simulink model "zad1b"  (R2016a)
settings: Solver=ode5  StartTime=0.0  StopTime=20  FixedStep=0.01  RelTol=1e-3
values from neighbouring files (symbols this model uses):
  b = 3    [zad1script.m]    (also in zad2script.m)
  kd = -b+2*m*ksi*omega    (= 1.2)    [zad1script.m]
  kp = m*omega^2    (= 9)    [zad1script.m]
  m = 1    [zad1script.m]    (also in zad2script.m)
  r = 4    [zad1script.m]
  sw = 1    [zad1script.m]
  swD = 1    [zad1script.m]    (also in zad2script.m)
settings Model: Creator=milos  LastModifiedBy=milos

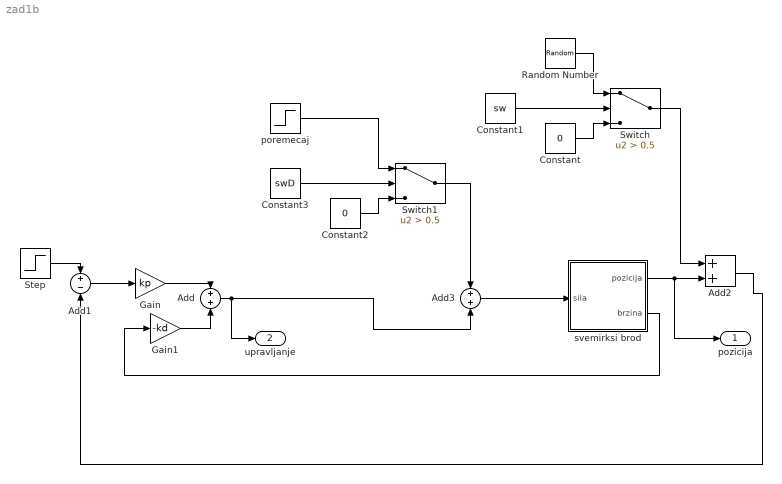
== system zad1b ==
  Add : Sum
  Add1 : Sum  Inputs=+-
  Add2 : Sum
  Add3 : Sum
  Constant : Constant  Value=0
  Constant1 : Constant  Value=sw
  Constant2 : Constant  Value=0
  Constant3 : Constant  Value=swD
  Gain : Gain  Gain=kp
  Gain1 : Gain  Gain=-kd
  Random Number : RandomNumber  Variance=0.01
  Step : Step  Time=0  After=r  SampleTime=0
  Switch : Switch  Criteria=u2 > Threshold  Threshold=0.5
  Switch1 : Switch  Criteria=u2 > Threshold  Threshold=0.5
  poremecaj : Step  After=3  SampleTime=0
  svemirksi brod : Subsystem
  pozicija : Outport
  upravljanje : Outport  Port=2
  wires:
  Gain1/1 -> Add/2
  Add/1 -> Add3/2, upravljanje/1
  Gain/1 -> Add/1
  Add1/1 -> Gain/1
  Step/1 -> Add1/1
  svemirksi brod/2(brzina) -> Gain1/1
  Random Number/1 -> Switch/1
  Constant/1 -> Switch/3
  Constant1/1 -> Switch/2
  Switch/1 -> Add2/1
  svemirksi brod/1(pozicija) -> pozicija/1, Add2/2
  Add2/1 -> Add1/2
  poremecaj/1 -> Switch1/1
  Constant2/1 -> Switch1/3
  Constant3/1 -> Switch1/2
  Add3/1 -> svemirksi brod/1(sila)
  Switch1/1 -> Add3/1

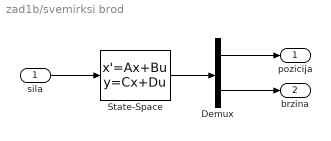
== system zad1b/svemirksi brod ==
  sila : Inport
  Demux : Demux  Outputs=2
  State-Space : StateSpace  A=[0 1;0 -b/m]  B=[0;1/m]  C=[1 0; 0 1]  D=[0;0]  X0=0
  pozicija : Outport
  brzina : Outport  Port=2
  wires:
  State-Space/1 -> Demux/1
  sila/1 -> State-Space/1
  Demux/1 -> pozicija/1
  Demux/2 -> brzina/1
